simulink model "gtcs_math_v2_r22a"  (R2022b)
settings: Solver=VariableStepAuto  StartTime=0.0  StopTime=10  RelTol=1e-3
undefined symbols (not defined in the file or in its folder): B_load, B_motor, B_reducer, GearRatio, J_load, J_motor, J_reducer, ke, kt, L_motor, R_motor
libraries: slpidlib x1, simulink x1
settings Model: DataDictionary=gtcs_math_v1.sldd  Creator=yusuf.ogut  LastModifiedBy=Yusuf
settings ModelReferenceCC: EnableRefExpFcnMdlSchedulingChecks=on

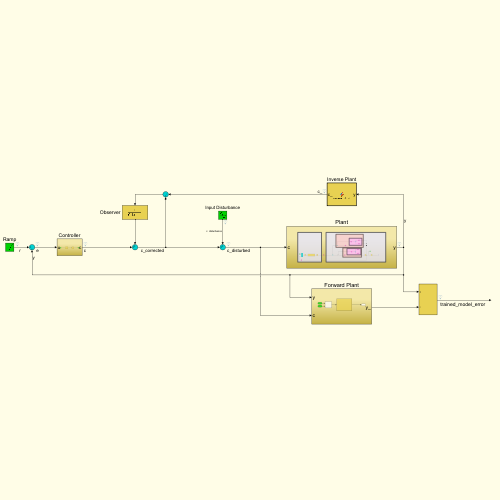
[thumbnail: Simulink's stored preview of the top-level diagram]
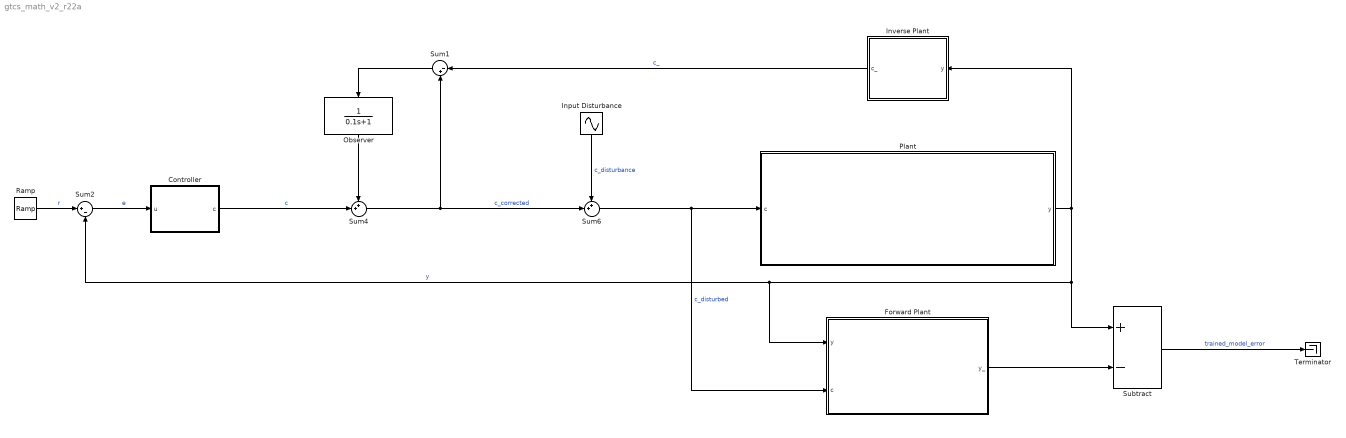
== system gtcs_math_v2_r22a ==
  Controller : Subsystem
  Forward Plant : Subsystem
  Input Disturbance : Sin  SampleTime=0
  Inverse Plant : MATLAB Function  TreatAsAtomicUnit=on
  Observer : TransferFcn  Denominator=[0.1 1]
  Plant : Subsystem
  Ramp : simulink/Sources/Ramp  slope=30  start=0  InitialOutput=0
  Subtract : Sum  Inputs=+-
  Sum1 : Sum  Inputs=|-+
  Sum2 : Sum  Inputs=|+-
  Sum4 : Sum  Inputs=++|
  Sum6 : Sum  Inputs=++|
  Terminator : Terminator
  wires:
  Plant/1(y) -> Inverse Plant/1(y), Forward Plant/1(y), Sum2/2, Subtract/1  "y"
  Sum2/1 -> Controller/1(u)  "e"
  Sum6/1 -> Forward Plant/2(c), Plant/1(c)  "c_disturbed"
  Ramp/1 -> Sum2/1  "r"
  Controller/1(c) -> Sum4/2  "c"
  Sum4/1 -> Sum6/2, Sum1/2  "c_corrected"
  Input Disturbance/1 -> Sum6/1  "c_disturbance"
  Inverse Plant/1(c_) -> Sum1/1  "c_"
  Sum1/1 -> Observer/1
  Observer/1 -> Sum4/1
  Forward Plant/1(y_) -> Subtract/2
  Subtract/1 -> Terminator/1  "trained_model_error"

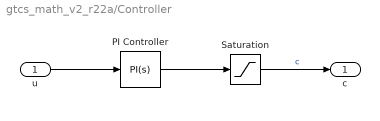
== system gtcs_math_v2_r22a/Controller ==
  u : Inport
  PI Controller : slpidlib/PID Controller  Controller=PI  Form=Parallel  TimeDomain=Continuous-time  UseExternalTs=off  SampleTime=-1  IntegratorMethod=Forward Euler  FilterMethod=Forward Euler  ControllerParametersSource=internal  P=1  I=0.12  UseKiTs=off  D=0  N=100  UseFilter=on  TunerSelectOption=Transfer Function Based (PID Tuner App)  InitialConditionSource=internal  InitialConditionForIntegrator=0  InitialConditionForFilter=0  DifferentiatorICPrevScaledInput=0  ExternalReset=none  TrackingMode=off  Kt=1  LimitOutput=off  SatLimitsSource=internal  UpperSaturationLimit=inf  LowerSaturationLimit=-inf  LinearizeAsGain=on  AntiWindupMode=none  Kb=1  LimitIntegrator=off  UpperIntegratorSaturationLimit=inf  LowerIntegratorSaturationLimit=-inf  POutMin=[]  POutMax=[]  IOutMin=[]  IOutMax=[]  DOutMin=[]  DOutMax=[]  NOutMin=[]  NOutMax=[]  SumOutMin=[]  SumOutMax=[]  SaturationOutMin=[]  SaturationOutMax=[]  PParamMin=[]  PParamMax=[]  IParamMin=[]  IParamMax=[]  DParamMin=[]  DParamMax=[]  NParamMin=[]  NParamMax=[]  KbParamMin=[]  KbParamMax=[]  KtParamMin=[]  KtParamMax=[]  KbOutMin=[]  KbOutMax=[]  KtOutMin=[]  KtOutMax=[]  IntegratorOutMin=[]  IntegratorOutMax=[]  FilterOutMin=[]  FilterOutMax=[]  SumI1OutMin=[]  SumI1OutMax=[]  SumI2OutMin=[]  SumI2OutMax=[]  SumI3OutMin=[]  SumI3OutMax=[]  SumI4OutMin=[]  SumI4OutMax=[]  SumDOutMin=[]  SumDOutMax=[]  DifferentiatorOutMin=[]  DifferentiatorOutMax=[]  FilterDiffOutCoefMin=[]  FilterDiffOutCoefMax=[]  ReciprocalOutMin=[]  ReciprocalOutMax=[]  SumDenOutMin=[]  SumDenOutMax=[]  SumNumOutMin=[]  SumNumOutMax=[]  DivideOutMin=[]  DivideOutMax=[]  UdiffTsProdOutMin=[]  UdiffTsProdOutMax=[]  NTsProdOutMin=[]  NTsProdOutMax=[]  UintegralTsProdOutMin=[]  UintegralTsProdOutMax=[]  UngainTsProdOutMin=[]  UngainTsProdOutMax=[]  ClampingZeroOutDataTypeStr=Inherit: Inherit via back propagation  ClampingZeroOutMin=[]  ClampingZeroOutMax=[]  FilterDenConstantOutDataTypeStr=Inherit: Inherit via back propagation  FilterDenConstantOutMin=[]  FilterDenConstantOutMax=[]  PCopyOutDataTypeStr=Inherit: Inherit via back propagation  PCopyOutMin=[]  PCopyOutMax=[]  NCopyOutDataTypeStr=Inherit: Inherit via back propagation  NCopyOutMin=[]  NCopyOutMax=[]  IntegratorContinuousStateAttributes=''  IntegratorStateMustResolveToSignalObject=off  IntegratorRTWStateStorageClass=Auto  FilterContinuousStateAttributes=''  FilterStateMustResolveToSignalObject=off  FilterRTWStateStorageClass=Auto  ParallelPVariant=InternalParameters  IdealPVariant=Disabled  IVariant=InternalParameters  DVariant=Disabled  IntegratorVariant=Continuous  SatVariant=Disabled  AWVariant=Passthrough  PCopyVariant=Disabled  TRVariant=Disabled  FdbkBlocksVariant=Forward  IdealPFdbkVariant=Disabled  SatFdbkVariant=Disabled  DerivativeFilterVariant=Disabled  NVariant=Disabled  NCopyVariant=Disabled_SignalSpec  FilterICVariant=Disabled  IntegratorICVariant=InternalICs  ExternalResetVariant=Disabled  TRSumVariant=Passthrough  SumFdbkVariant=Disabled  SumVariant=Sum_PI  TsampFilterVariant=InternalTs  TsampNgainVariant=Passthrough  TsampIntegralVariant=Passthrough  ExternalSaturationOutDataTypeStr=Inherit: Same as second input
  Saturation : Saturate  UpperLimit=28  LowerLimit=-28
  c : Outport
  wires:
  Saturation/1 -> c/1  "c"
  PI Controller/1 -> Saturation/1
  u/1 -> PI Controller/1

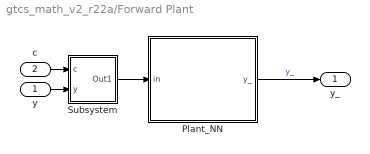
== system gtcs_math_v2_r22a/Forward Plant ==
  y : Inport
  c : Inport  Port=2
  Plant_NN : MATLAB Function  TreatAsAtomicUnit=on
  Subsystem : Subsystem
  y_ : Outport
  wires:
  Subsystem/1(Out1) -> Plant_NN/1(in)
  Plant_NN/1(y_) -> y_/1  "y_"
  c/1 -> Subsystem/1(c)
  y/1 -> Subsystem/2(y)

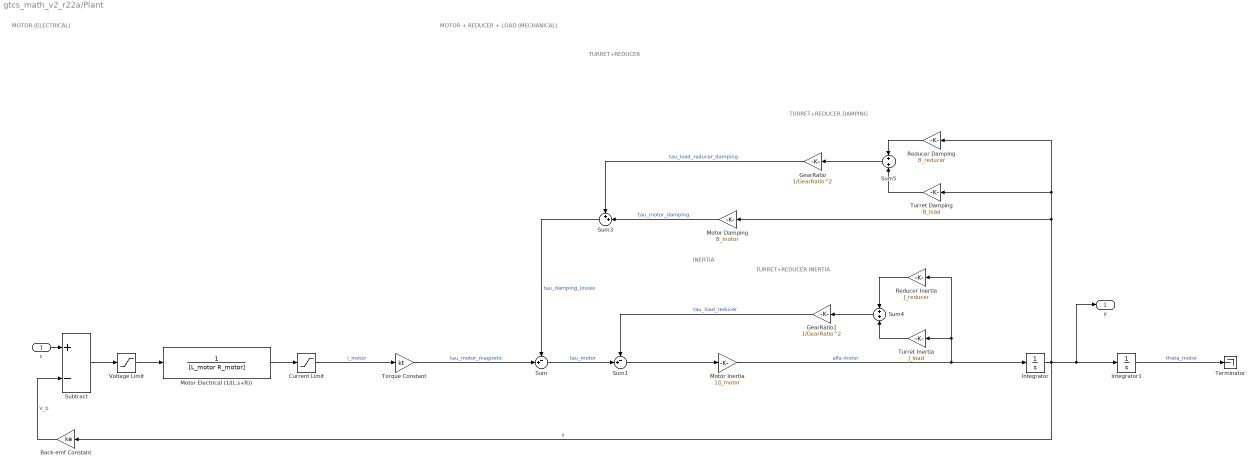
== system gtcs_math_v2_r22a/Plant ==
  note: TURRET+REDUCER INERTIA
  note: TURRET+REDUCER DAMPING
  note: TURRET+REDUCER
  note: INERTIA
  note: MOTOR (ELECTRICAL)
  note: MOTOR + REDUCER + LOAD (MECHANICAL)
  c : Inport
  Back-emf Constant : Gain  Gain=ke
  Current Limit : Saturate  UpperLimit=80  LowerLimit=-80
  GearRatio : Gain  Gain=1/GearRatio^2
  GearRatio1 : Gain  Gain=1/GearRatio^2
  Integrator : Integrator
  Integrator1 : Integrator
  Motor Damping : Gain  Gain=B_motor
  Motor Electrical (1/(L.s+R)) : TransferFcn  Denominator=[L_motor R_motor]
  Motor Inertia : Gain  Gain=1/J_motor
  Reducer Damping : Gain  Gain=B_reducer
  Reducer Inertia : Gain  Gain=J_reducer
  Subtract : Sum  Inputs=+-
  Sum : Sum  Inputs=-+|
  Sum1 : Sum  Inputs=-+|
  Sum3 : Sum  Inputs=++|
  Sum4 : Sum
  Sum5 : Sum
  Terminator : Terminator
  Torque Constant : Gain  Gain=kt
  Turret Damping : Gain  Gain=B_load
  Turret Inertia : Gain  Gain=J_load
  Voltage Limit : Saturate  UpperLimit=28  LowerLimit=-28
  y : Outport
  wires:
  Turret Damping/1 -> Sum5/2
  Reducer Inertia/1 -> Sum4/1
  Torque Constant/1 -> Sum/2  "tau_motor_magnetic"
  GearRatio/1 -> Sum3/1  "tau_load_reducer_damping"
  Integrator/1 -> y/1, Integrator1/1, Back-emf Constant/1, Turret Damping/1, Reducer Damping/1, Motor Damping/1  "y"
  Current Limit/1 -> Torque Constant/1  "i_motor"
  Sum3/1 -> Sum/1  "tau_damping_losses"
  Motor Inertia/1 -> Integrator/1, Turret Inertia/1, Reducer Inertia/1  "alfa motor"
  Sum1/1 -> Motor Inertia/1
  GearRatio1/1 -> Sum1/1  "tau_load_reducer"
  Integrator1/1 -> Terminator/1  "theta_motor"
  Turret Inertia/1 -> Sum4/2
  Sum5/1 -> GearRatio/1
  Sum/1 -> Sum1/2  "tau_motor"
  Motor Damping/1 -> Sum3/2  "tau_motor_damping"
  Voltage Limit/1 -> Motor Electrical (1/(L.s+R))/1
  Back-emf Constant/1 -> Subtract/2  "V_b"
  c/1 -> Subtract/1
  Motor Electrical (1/(L.s+R))/1 -> Current Limit/1
  Subtract/1 -> Voltage Limit/1
  Sum4/1 -> GearRatio1/1
  Reducer Damping/1 -> Sum5/1

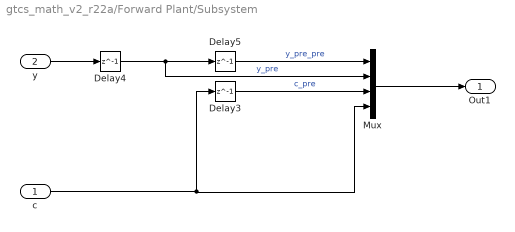
== system gtcs_math_v2_r22a/Forward Plant/Subsystem ==
  c : Inport
  y : Inport  Port=2
  Delay3 : Delay  DelayLength=1  SampleTime=0.01
  Delay4 : Delay  DelayLength=1  SampleTime=0.01
  Delay5 : Delay  DelayLength=1  SampleTime=0.01
  Mux : Mux
  Out1 : Outport
  wires:
  c/1 -> Mux/4, Delay3/1
  Delay4/1 -> Delay5/1, Mux/2  "y_pre"
  Delay3/1 -> Mux/3  "c_pre"
  Mux/1 -> Out1/1
  Delay5/1 -> Mux/1  "y_pre_pre"
  y/1 -> Delay4/1

== matlab function gtcs_math_v2_r22a/Inverse Plant ==
  data: y input; c_ output
function c_ = inverse_plant(y)
    y_ =  0.0534; r_ = 16.0258;
    c__ = 1.2811; r__ = 384.4721;
    input_training = (y - c__)/r__;
%     Phi = [ -0.7229   -0.1132         0         0
%             -0.7229   -0.1132         0         0
%             -0.7229   -0.1132         0         0
%             -0.4882   -0.4882   -0.4882   -0.1223];
    Phi = [    0.9934    0.0476    0.4243    0.7847
    0.8882    0.5768    0.4609    0.4714
    0.2196   -0.3380    0.7702    0.0358
    0.6646    0.3821    0.3627   -0.0466];
    BIAS = -.1;
    % FORWARD PASS:
    NUM_INP = 1; NUM_HID = 3;
    input_vector = [input_training;BIAS];
    S1 = Phi(1:NUM_HID,1:NUM_INP+1)*input_vector;
    O1 = tanh(S1);
    S2 = Phi(NUM_HID+1:end,1:NUM_HID+1)*[O1;BIAS];
    c_ = S2*r_+y_;
end

== matlab function gtcs_math_v2_r22a/Forward Plant/Plant_NN ==
  data: in input; y_ output
function y_ = forward_pass(in)
    c_sf_i_4 = 0.0534;     r_sf_i_4 = 16.0258;
    c_sf_i_3 = 0.0534;     r_sf_i_3 = 16.0258;
    c_sf_i_2 = 1.2811;     r_sf_i_2 = 384.4721;
    c_sf_i_1 = 1.2811;     r_sf_i_1 = 384.4721;
    c_sf_o_1 = 1.28114;    r_sf_o_1 = 384.4721;
    input_training = (([in(4) in(3) in(2) in(1)] - [c_sf_i_4 c_sf_i_3 c_sf_i_2 c_sf_i_1]) ./ [r_sf_i_4 r_sf_i_3 r_sf_i_2 r_sf_i_1])';

    Phi = [   -0.1896   -0.1745   -0.1475   -0.1324   -0.0377         0         0         0         0         0         0
   -0.1896   -0.1745   -0.1475   -0.1324   -0.0377         0         0         0         0         0         0
   -0.1896   -0.1745   -0.1475   -0.1324   -0.0377         0         0         0         0         0         0
   -0.1896   -0.1745   -0.1475   -0.1324   -0.0377         0         0         0         0         0         0
   -0.1896   -0.1745   -0.1475   -0.1324   -0.0377         0         0         0         0         0         0
   -0.1896   -0.1745   -0.1475   -0.1324   -0.0377         0         0         0         0         0         0
   -0.1896   -0.1745   -0.1475   -0.1324   -0.0377         0         0         0         0         0         0
   -0.1896   -0.1745   -0.1475   -0.1324   -0.0377         0         0         0         0         0         0
   -0.1896   -0.1745   -0.1475   -0.1324   -0.0377         0         0         0         0         0         0
   -0.1896   -0.1745   -0.1475   -0.1324   -0.0377         0         0         0         0         0         0
   -0.1605   -0.1605   -0.1605   -0.1605   -0.1605   -0.1605   -0.1605   -0.1605   -0.1605   -0.1605   -0.0594];

    BIAS = -.1;
    % FORWARD PASS:
    NUM_INP = 4; NUM_HID = 10;
    input_vector = [input_training;BIAS];
    S1 = Phi(1:NUM_HID,1:NUM_INP+1)*input_vector;
    O1 = tanh(S1);
    S2 = Phi(NUM_HID+1:end,1:NUM_HID+1)*[O1;BIAS];
    y_ = S2 * r_sf_o_1 + c_sf_o_1;
end
